simulink model "Comm_gatera"  (R2020a)
settings: Solver=VariableStepAuto  StartTime=0.0  StopTime=20  RelTol=1e-3
settings Model: DataDictionary=Registro_variables.sldd  Creator=Juan  LastModifiedBy=Juan

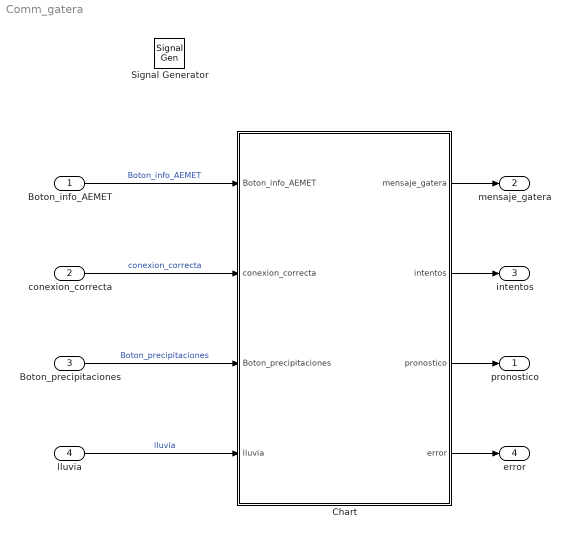
== system Comm_gatera ==
  Boton_info_AEMET : Inport  OutMin=0  OutMax=1  OutDataTypeStr=boolean  PortDimensions=1
  conexion_correcta : Inport  Port=2  OutMin=0  OutMax=1  OutDataTypeStr=boolean  PortDimensions=1
  Boton_precipitaciones : Inport  Port=3  OutMin=0  OutMax=1  OutDataTypeStr=boolean  PortDimensions=1
  lluvia : Inport  Port=4  OutMin=0  OutMax=10  OutDataTypeStr=double  PortDimensions=1
  Chart : Stateflow chart  TreatAsAtomicUnit=on
  pronostico : Outport  SignalName=pronostico  OutMin=0  OutMax=1  OutDataTypeStr=boolean  PortDimensions=1  VectorParamsAs1DForOutWhenUnconnected=off
      settings: MustResolveToSignalObject=on
  mensaje_gatera : Outport  Port=2  SignalName=mensaje_gatera  OutMin=0  OutMax=30  OutDataTypeStr=double  PortDimensions=1  VectorParamsAs1DForOutWhenUnconnected=off
      settings: MustResolveToSignalObject=on
  intentos : Outport  Port=3  SignalName=intentos  OutMin=0  OutMax=30  OutDataTypeStr=double  PortDimensions=1  VectorParamsAs1DForOutWhenUnconnected=off
      settings: MustResolveToSignalObject=on
  error : Outport  Port=4  SignalName=error  OutMin=0  OutMax=1  OutDataTypeStr=double  PortDimensions=1  VectorParamsAs1DForOutWhenUnconnected=off
      settings: MustResolveToSignalObject=on
  Signal Generator : SignalGenerator  IOType=siggen
  wires:
  Boton_info_AEMET/1 -> Chart/1(Boton_info_AEMET)  "Boton_info_AEMET"
  conexion_correcta/1 -> Chart/2(conexion_correcta)  "conexion_correcta"
  Boton_precipitaciones/1 -> Chart/3(Boton_precipitaciones)  "Boton_precipitaciones"
  lluvia/1 -> Chart/4(lluvia)  "lluvia"
  Chart/1(mensaje_gatera) -> mensaje_gatera/1
  Chart/3(pronostico) -> pronostico/1
  Chart/2(intentos) -> intentos/1
  Chart/4(error) -> error/1

== stateflow chart Comm_gatera/Chart ==
  state INICIO1
    pronostico = false
    intentos = 0
    mensaje_gatera = 0
    error = 0
  state ERROR_CONEXION
    intentos = 0
    pronostico = false
    error = 1
  state ACCESO_METEOROLOGIA
    state MENSAJE_ENVIADO
      mensaje_gatera = 0
    state CONEXION_INTERNET
      pronostico = false
      intentos = intentos + 1
    state PUBLICAR_ALERTA_API
      mensaje_gatera = 1
    state PUBLICAR_NO_ALERTA_API
      mensaje_gatera = 2
    state PARTE_METEORLOGICO
      pronostico = true
      intentos = 0
    state COMPROBACION_PRECIPITACIONES
      pronostico = false
    (default) -> CONEXION_INTERNET
    PUBLICAR_ALERTA_API -> MENSAJE_ENVIADO : [lluvia == 1]
    PUBLICAR_NO_ALERTA_API -> MENSAJE_ENVIADO : [lluvia == 2]
    CONEXION_INTERNET -> CONEXION_INTERNET [order 1] : [~conexion_correcta && intentos<30]
    CONEXION_INTERNET -> PARTE_METEORLOGICO [order 3] : [conexion_correcta]
    PARTE_METEORLOGICO -> PARTE_METEORLOGICO [order 2] : [~Boton_precipitaciones]
    COMPROBACION_PRECIPITACIONES -> PUBLICAR_ALERTA_API [order 1] : [lluvia == 1]
    COMPROBACION_PRECIPITACIONES -> PUBLICAR_NO_ALERTA_API [order 2] : [lluvia == 2]
    COMPROBACION_PRECIPITACIONES -> COMPROBACION_PRECIPITACIONES [order 3] : [lluvia == 0]
    PARTE_METEORLOGICO -> COMPROBACION_PRECIPITACIONES [order 1] : [Boton_precipitaciones]
  (default) -> INICIO1
  INICIO1 -> INICIO1 [order 1] : [~Boton_info_AEMET]
  ERROR_CONEXION -> INICIO1 : [intentos == 0]
  INICIO1 -> ACCESO_METEOROLOGIA [order 2] : [Boton_info_AEMET]
  CONEXION_INTERNET -> ERROR_CONEXION [order 2] : [intentos>30]
  data: Boton_info_AEMET input; conexion_correcta input; Boton_precipitaciones input; lluvia input; mensaje_gatera output; intentos output; pronostico output; error output
